simulink model "sim_linear_control_pos"  (R2018a)
settings: Solver=ode3  StartTime=0.0  StopTime=t(end)  FixedStep=dt  RelTol=1e-3
values from neighbouring files (symbols this model uses):
  A = [-(Cf+Cr)/(m*Vx)  -(a*Cf-b*Cr)/(m*Vx)-Vx ... (first row only)    [lin_control_pos.m]
  B = [Cf/m; a*Cf/Iz]    [lin_control_pos.m]
  C = Col(3,:)    [lin_control_pos.m]
  CA = C*Aol    [lin_control_pos.m]
  fc = 0.5    [lin_control_pos.m]
  invCB = pinv(C*Bol)    [lin_control_pos.m]
  K_ay = 8    [lin_control_pos.m]
  K_Vy = 4    [lin_control_pos.m]
  K_y = 2    [lin_control_pos.m]
  rho = 1/R    (= 0.0942477796077)    [lin_control_pos.m]
  t1 = 1    [lin_control_pos.m]
  t2 = 7    [lin_control_pos.m]
  Vx = 10/3.6    (= 2.77777777778)    [lin_control_pos.m]
  w = 10    [lin_control_pos.m]
settings Model: Creator=E183308  LastModifiedBy=E183308

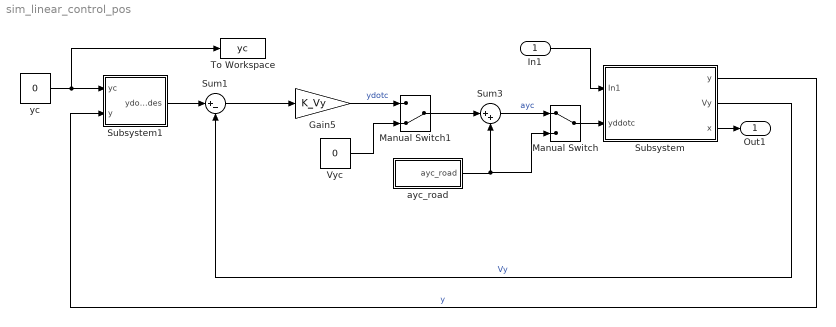
== system sim_linear_control_pos ==
  In1 : Inport
  Gain5 : Gain  Gain=K_Vy
  Manual Switch : ManualSwitch
  Manual Switch1 : ManualSwitch  CurrentSetting=0
  Subsystem : Subsystem
  Subsystem1 : Subsystem
  Sum1 : Sum  Inputs=|+-
  Sum3 : Sum  Inputs=|++
  To Workspace : ToWorkspace  VariableName=yc  SampleTime=-1
  Vyc : Constant  Value=0
  ayc_road : Subsystem
  yc : Constant  Value=0
  Out1 : Outport
  wires:
  Subsystem/2(Vy) -> Sum1/2  "Vy"
  In1/1 -> Subsystem/1(In1)
  Subsystem/3(x) -> Out1/1
  Subsystem1/1(ydot_des) -> Sum1/1
  Subsystem/1(y) -> Subsystem1/2(y)  "y"
  yc/1 -> Subsystem1/1(yc), To Workspace/1
  Sum3/1 -> Manual Switch/1  "ayc"
  ayc_road/1(ayc_road) -> Manual Switch/2, Sum3/2
  Manual Switch/1 -> Subsystem/2(yddotc)
  Sum1/1 -> Gain5/1
  Vyc/1 -> Manual Switch1/2
  Gain5/1 -> Manual Switch1/1  "ydotc"
  Manual Switch1/1 -> Sum3/1

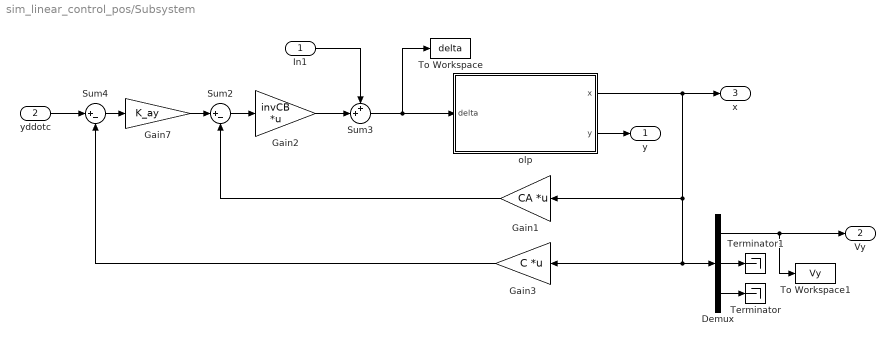
== system sim_linear_control_pos/Subsystem ==
  In1 : Inport
  yddotc : Inport  Port=2
  Demux : Demux  Outputs=[1 1 3]
  Gain1 : Gain  Gain=CA  Multiplication=Matrix(K*u)
  Gain2 : Gain  Gain=invCB  Multiplication=Matrix(K*u)
  Gain3 : Gain  Gain=C  Multiplication=Matrix(K*u)
  Gain7 : Gain  Gain=K_ay
  Sum2 : Sum  Inputs=|+-
  Sum3 : Sum  Inputs=++|
  Sum4 : Sum  Inputs=|+-
  Terminator : Terminator
  Terminator1 : Terminator
  To Workspace : ToWorkspace  VariableName=delta  SampleTime=-1
  To Workspace1 : ToWorkspace  VariableName=Vy  SampleTime=-1
  olp : Subsystem
  y : Outport
  Vy : Outport  Port=2
  x : Outport  Port=3
  wires:
  yddotc/1 -> Sum4/1
  Gain3/1 -> Sum4/2
  Sum2/1 -> Gain2/1
  Sum4/1 -> Gain7/1
  Gain1/1 -> Sum2/2
  Gain7/1 -> Sum2/1
  Gain2/1 -> Sum3/2
  Sum3/1 -> To Workspace/1, olp/1(delta)
  In1/1 -> Sum3/1
  olp/2(y) -> y/1
  Demux/3 -> Terminator/1
  Demux/1 -> To Workspace1/1, Vy/1
  olp/1(x) -> Demux/1, Gain3/1, Gain1/1, x/1
  Demux/2 -> Terminator1/1

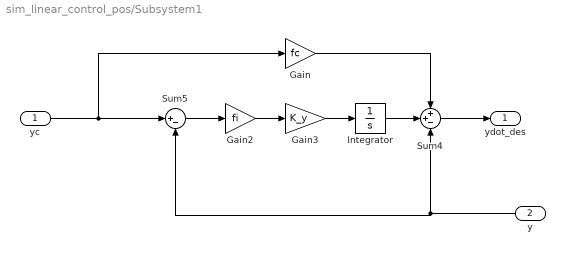
== system sim_linear_control_pos/Subsystem1 ==
  yc : Inport
  y : Inport  Port=2
  Gain : Gain  Gain=fc
  Gain2 : Gain  Gain=fi
  Gain3 : Gain  Gain=K_y
  Integrator : Integrator
  Sum4 : Sum  Inputs=++-
  Sum5 : Sum  Inputs=|+-
  ydot_des : Outport
  wires:
  Gain3/1 -> Integrator/1
  Sum4/1 -> ydot_des/1
  Gain2/1 -> Gain3/1
  Sum5/1 -> Gain2/1
  yc/1 -> Gain/1, Sum5/1
  Integrator/1 -> Sum4/2
  Gain/1 -> Sum4/1
  y/1 -> Sum5/2, Sum4/3

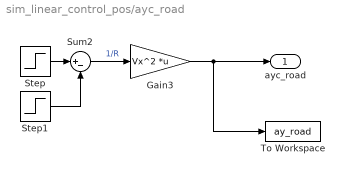
== system sim_linear_control_pos/ayc_road ==
  Gain3 : Gain  Gain=Vx^2  Multiplication=Matrix(K*u)
  Step : Step  Time=t1  After=rho  SampleTime=0
  Step1 : Step  Time=t2  After=rho  SampleTime=0
  Sum2 : Sum  Inputs=|+-
  To Workspace : ToWorkspace  VariableName=ay_road  SampleTime=-1
  ayc_road : Outport
  wires:
  Step1/1 -> Sum2/2
  Step/1 -> Sum2/1
  Sum2/1 -> Gain3/1  "1/R"
  Gain3/1 -> To Workspace/1, ayc_road/1

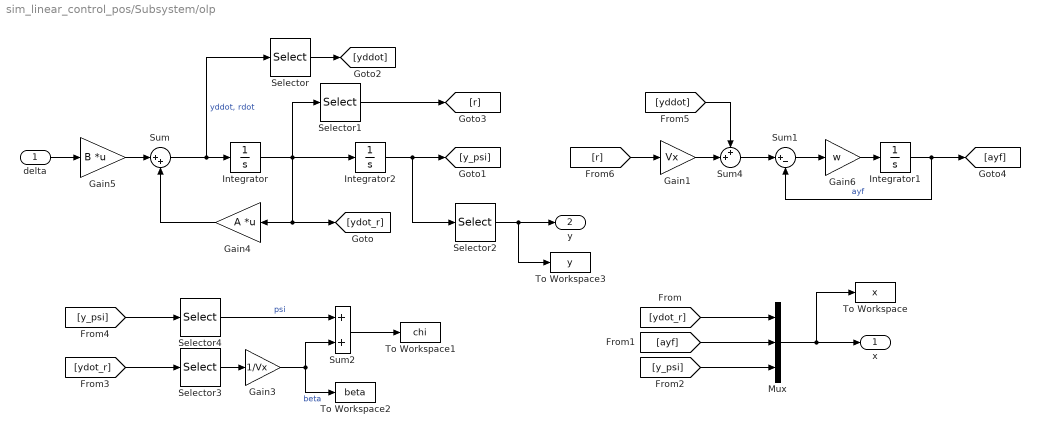
== system sim_linear_control_pos/Subsystem/olp ==
  delta : Inport
  Gain1 : Gain  Gain=Vx
  Gain3 : Gain  Gain=1/Vx
  Gain4 : Gain  Gain=A  Multiplication=Matrix(K*u)
  Gain5 : Gain  Gain=B  Multiplication=Matrix(K*u)
  Gain6 : Gain  Gain=w
  Integrator : Integrator  InitialCondition=[0;0]
  Integrator1 : Integrator
  Integrator2 : Integrator  InitialCondition=[0;0]
  Mux : Mux  Inputs=3
  Selector : Selector  InputPortWidth=2  IndexOptions=Index vector (dialog)  Indices=1  OutputSizes=1
  Selector1 : Selector  InputPortWidth=2  IndexOptions=Index vector (dialog)  Indices=2  OutputSizes=1
  Selector2 : Selector  InputPortWidth=2  IndexOptions=Index vector (dialog)  Indices=1  OutputSizes=1
  Selector3 : Selector  InputPortWidth=2  IndexOptions=Index vector (dialog)  Indices=1  OutputSizes=1
  Selector4 : Selector  InputPortWidth=2  IndexOptions=Index vector (dialog)  Indices=2  OutputSizes=1
  Sum : Sum  Inputs=|++
  Sum1 : Sum  Inputs=|+-
  Sum2 : Sum
  Sum4 : Sum  Inputs=++|
  To Workspace : ToWorkspace  VariableName=x  SampleTime=-1
  To Workspace1 : ToWorkspace  VariableName=chi  SampleTime=-1
  To Workspace2 : ToWorkspace  VariableName=beta  SampleTime=-1
  To Workspace3 : ToWorkspace  VariableName=y  SampleTime=-1
  x : Outport
  y : Outport  Port=2
  wires:
  Integrator/1 -> Selector1/1, Integrator2/1, [ydot_r], Gain4/1
  delta/1 -> Gain5/1
  Gain5/1 -> Sum/1
  Gain4/1 -> Sum/2
  Gain6/1 -> Integrator1/1
  Sum1/1 -> Gain6/1
  Mux/1 -> x/1, To Workspace/1
  Integrator1/1 -> [ayf], Sum1/2  "ayf"
  Sum/1 -> Selector/1, Integrator/1  "yddot, rdot"
  Gain1/1 -> Sum4/2
  Sum4/1 -> Sum1/1
  Selector3/1 -> Gain3/1
  Selector4/1 -> Sum2/1  "psi"
  Gain3/1 -> To Workspace2/1, Sum2/2  "beta"
  Sum2/1 -> To Workspace1/1
  [ydot_r] -> Mux/1
  [ayf] -> Mux/2
  [y_psi] -> Mux/3
  [ydot_r] -> Selector3/1
  [y_psi] -> Selector4/1
  Integrator2/1 -> Selector2/1, [y_psi]
  Selector/1 -> [yddot]
  [yddot] -> Sum4/1
  Selector1/1 -> [r]
  [r] -> Gain1/1
  Selector2/1 -> To Workspace3/1, y/1
